simulink model "mpc_2"  (R2021a)
settings: Solver=FixedStepAuto  StartTime=0.0  StopTime=10  FixedStep=0.002  RelTol=1e-6  AbsTol=1e-9
settings Model: Creator=dell  LastModifiedBy=dell

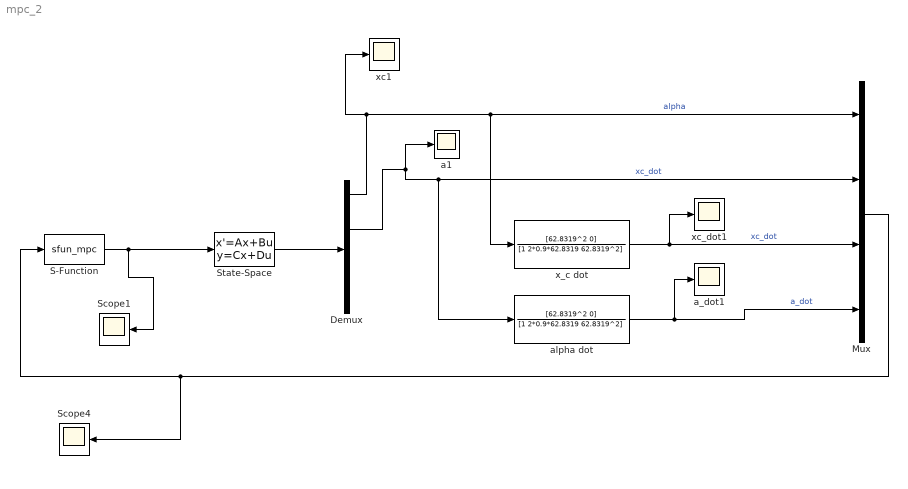
== system mpc_2 ==
  Demux : Demux
  Mux : Mux
  S-Function : S-Function  FunctionName=sfun_mpc  Parameters=pa  SFunctionDeploymentMode=off  EnableBusSupport=off
  Scope1 : Scope
  Scope4 : Scope
  State-Space : StateSpace  A=|  B=[ 0 ;0 ;1.5662 ;6.7834]  C=[1 0 0 0;0 1 0 0;0 0 1 0;0 0 0 1]  D=[0;0;0;0]  InitialCondition=[0;0.1;0;0]
      | [0   0        0        1     ;
      |         0   0        1        0     ;
      |         0   0.8703   -11.924 -0.0094;
      |         0   46.2580 -51.6449  -0.5012 ]
  a1 : Scope
  a_dot1 : Scope
  alpha dot : TransferFcn  Numerator=[62.8319^2 0]  Denominator=[1 2*0.9*62.8319 62.8319^2]
  x_c dot : TransferFcn  Numerator=[62.8319^2 0]  Denominator=[1 2*0.9*62.8319 62.8319^2]
  xc1 : Scope
  xc_dot1 : Scope
  wires:
  Mux/1 -> Scope4/1, S-Function/1
  Demux/1 -> x_c dot/1, Mux/1, xc1/1  "alpha"
  State-Space/1 -> Demux/1
  Demux/2 -> alpha dot/1, Mux/2, a1/1  "xc_dot"
  x_c dot/1 -> xc_dot1/1, Mux/3  "xc_dot"
  alpha dot/1 -> a_dot1/1, Mux/4  "a_dot"
  S-Function/1 -> State-Space/1, Scope1/1
